simulink model "UpdatedAttitudeSim"  (R2023b)
settings: Solver=FixedStepAuto  StartTime=0.0  StopTime=tf  FixedStep=tstep  RelTol=1e-3  EnableMultiTasking=on
values from neighbouring files (symbols this model uses):
  C = [1 0 0 0 0 0;     0 1 0 0 0 0;     0 0 1 0 0 0]    [Attitude.m]    (also in Translational.m = eye(6); UpdatedAttitude.m = [1 0 0 0 0 0;      0 1 0 0 0 0;      0 0 1 0 0 0])
  I = [Ixx,Iyy,Izz]    [Attitude.m]    (also in UpdatedAttitude.m = eye(3))
  M = [0.1;0.2;0.3]    [UpdatedAttitude.m]
  P0 = zeros(3,3)    [UpdatedAttitude.m]
  Q = 500.*diag([1 1 1 0 0 0 0 0 0])    [Attitude.m]    (also in Filter.m = dt^2.*ones(3,3); Translational.m = diag([1 1 10 0 0 0 0 0 0]); UpdatedAttitude.m = G*G')
  R = eye(3)    [Attitude.m]    (also in Filter.m; Translational.m = diag([1 2000 2000 2000]); UpdatedAttitude.m)
  Ref = out.Reference.signals.values    [Attitude.m]    (also in main.m = out.Ref.signals.values)
  tstep = 0.001    [ActuatorModel.m]    (also in Attitude.m; Translational.m; UpdatedAttitude.m = 0.0001; main.m)
  x0 = [0; 0; 0]    [UpdatedAttitude.m]    (also in main.m = [0;0;0;0;0;0;0;0;0;0;0;0])
libraries: simulink x1
settings Model: Creator=Nathan Dablain  LastModifiedBy=Nathan Dablain

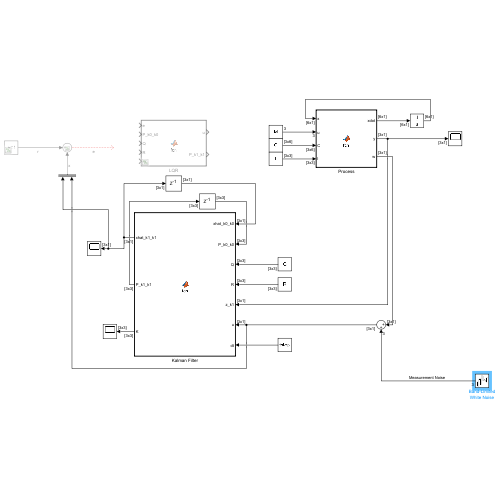
[thumbnail: Simulink's stored preview of the top-level diagram]
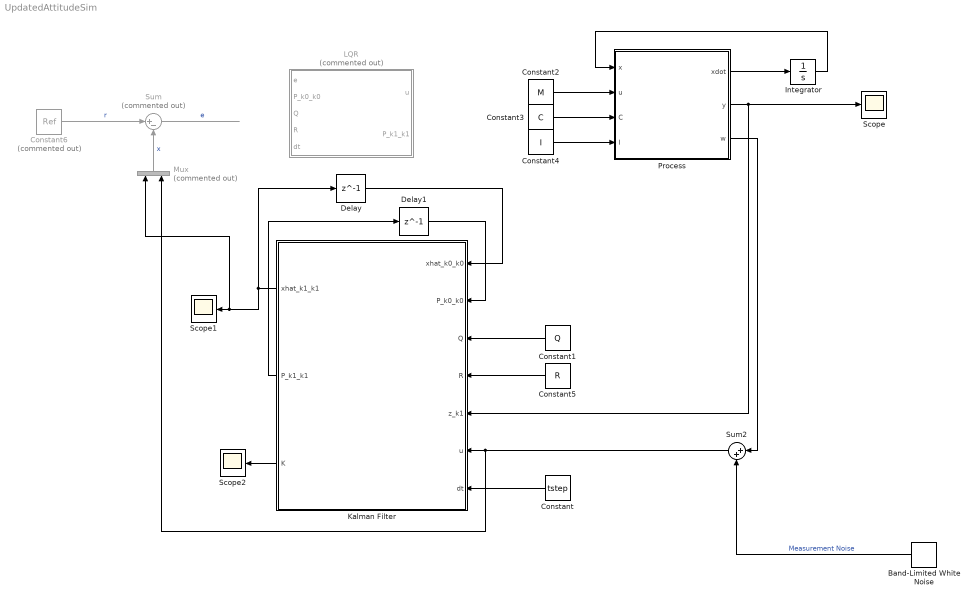
== system UpdatedAttitudeSim ==
  Band-Limited White Noise : simulink/Sources/Band-Limited White Noise  Cov=[3 3 3].*0.001  Ts=tstep  seed=[23341]
  Constant : Constant  Value=tstep
  Constant1 : Constant  Value=Q
  Constant2 : Constant  Value=M
  Constant3 : Constant  Value=C
  Constant4 : Constant  Value=I
  Constant5 : Constant  Value=R
  Constant6 : Constant  Commented=on  Value=Ref
  Delay : Delay  DelayLength=1  InitialCondition=x0
  Delay1 : Delay  DelayLength=1  InitialCondition=P0
  Integrator : Integrator  InitialCondition=zeros(6,1)
  Kalman Filter : MATLAB Function  TreatAsAtomicUnit=on
  LQR : MATLAB Function  Commented=on  TreatAsAtomicUnit=on
  Mux : Mux  Commented=on  Inputs=2
  Process : MATLAB Function  TreatAsAtomicUnit=on
  Scope : Scope
  Scope1 : Scope
  Scope2 : Scope
  Sum : Sum  Commented=on  Inputs=|+-
  Sum2 : Sum  Inputs=|++
  wires:
  Kalman Filter/1(xhat_k1_k1) -> Mux/1, Scope1/1, Delay/1
  Kalman Filter/2(P_k1_k1) -> Delay1/1
  Delay/1 -> Kalman Filter/1(xhat_k0_k0)
  Delay1/1 -> Kalman Filter/2(P_k0_k0)
  Constant/1 -> Kalman Filter/7(dt)
  Constant1/1 -> Kalman Filter/3(Q)
  Process/2(y) -> Scope/1, Kalman Filter/5(z_k1)
  Process/1(xdot) -> Integrator/1
  Integrator/1 -> Process/1(x)
  Constant2/1 -> Process/2(u)
  Constant3/1 -> Process/3(C)
  Constant4/1 -> Process/4(I)
  Process/3(w) -> Sum2/1
  Band-Limited White Noise/1 -> Sum2/2  "Measurement Noise"
  Sum2/1 -> Kalman Filter/6(u), Mux/2
  Constant5/1 -> Kalman Filter/4(R)
  Mux/1 -> Sum/2  "x"
  Constant6/1 -> Sum/1  "r"
  Sum/1 -> ?  "e"
  Kalman Filter/3(K) -> Scope2/1

== matlab function UpdatedAttitudeSim/Kalman Filter ==
  data: xhat_k0_k0 input; P_k0_k0 input; Q input; R input; z_k1 input; xhat_k1_k1 output; u input; dt input; P_k1_k1 output; K output
function [xhat_k1_k1,P_k1_k1,K] = fcn(xhat_k0_k0,P_k0_k0,Q,R,z_k1,u,dt)
% xhat = [phi       theta     psi]
% u = [wx       wy      wz]
H = eye(3);
phi = xhat_k0_k0(1);
theta = xhat_k0_k0(2);
% Treat gyro output as input to filter
F = eye(3); % Discretized state transition matrix
B = [1 sin(phi)*tan(theta) cos(phi)*tan(theta);...
     0 cos(phi)            -sin(phi);...
     0 sin(phi)*sec(theta) cos(phi)*sec(theta)].*dt; % Discretized control input model
xhat_k1_k0 = F*xhat_k0_k0 + B*u;
P_k1_k0 = F*P_k0_k0*F' + Q;
ybar_k0 = z_k1-(H*xhat_k1_k0); % Initial residual
S = H*P_k1_k0*H' + R;
K = P_k1_k0*H'*inv(S);
xhat_k1_k1 = xhat_k1_k0 + K*ybar_k0;
P_k1_k1 = (eye(3)-K*H)*P_k1_k0;
end

== matlab function UpdatedAttitudeSim/Process ==
  data: x input; xdot output; u input; y output; C input; I input; w output
function [xdot,y,w] = fcn(x,u,C,I)
%
xdot = [[1 sin(x(1))*tan(x(2)) cos(x(1))*tan(x(2));...
    0 cos(x(1)) -sin(x(1));...
    0 sin(x(1))*sec(x(2)) cos(x(1))*sec(x(2))]*x(4:6);...
    I\(u - cross(x(4:6),I*x(4:6)))];
y = C*x;
w = x(4:6);
end

== matlab function UpdatedAttitudeSim/LQR ==
  data: e input; P_k0_k0 input; Q input; R input; u output; dt input; P_k1_k1 output
function [u,P_k1_k1] = fcn(e,P_k0_k0,Q,R,dt)
% xhat = [phi       theta     psi]
% u = [wx       wy      wz]
H = eye(3);
phi = xhat_k0_k0(1);
theta = xhat_k0_k0(2);
% Treat gyro output as input to filter
F = eye(3); % Discretized state transition matrix
B = [1 sin(phi)*tan(theta) cos(phi)*tan(theta);...
     0 cos(phi)            -sin(phi);...
     0 sin(phi)*sec(theta) cos(phi)*sec(theta)].*dt; % Discretized control input model
P_k1_k0 = F*P_k0_k0*F' + Q;
S = H*P_k1_k0*H' + R;
K = P_k1_k0*H'*inv(S);
P_k1_k1 = (eye(3)-K*H)*P_k1_k0;
u = K*e;
end
